simulink model "p3"  (R2020a)
settings: Solver=VariableStepAuto  StartTime=0.0  StopTime=10  RelTol=1e-3
model workspace (MAT data in the model file):
  A = Simulink.Parameter
  A.Value = 0.5792
  A.DataType = 'auto'
  A.Dimensions = [1 1]
  B = Simulink.Parameter
  B.Value = -1
  B.DataType = 'auto'
  B.Dimensions = [1 1]
  C = Simulink.Parameter
  C.Value = 1
  C.DataType = 'auto'
  C.Dimensions = [1 1]
  D = Simulink.Parameter
  D.Value = 0.1584
  D.DataType = 'auto'
  D.Dimensions = [1 1]
settings Model: Creator=007  LastModifiedBy=007

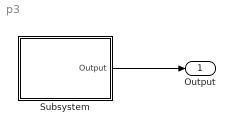
== system p3 ==
  Subsystem : Subsystem
  Output : Outport
  wires:
  Subsystem/1(Output) -> Output/1

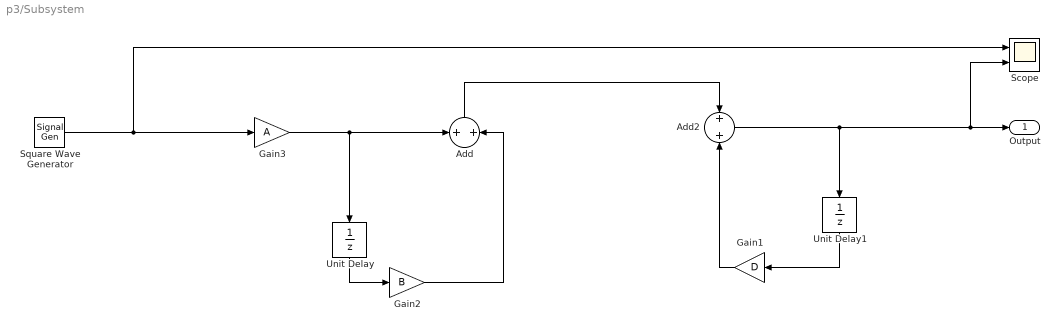
== system p3/Subsystem ==
  Add : Sum
  Add2 : Sum
  Gain1 : Gain  Gain=D
  Gain2 : Gain  Gain=B
  Gain3 : Gain  Gain=A
  Scope : Scope  NumInputPorts=2
  Square Wave Generator : SignalGenerator  WaveForm=square  Frequency=10  Units=rad/sec
  Unit Delay : UnitDelay  SampleTime=-1  HasFrameUpgradeWarning=on
  Unit Delay1 : UnitDelay  SampleTime=-1  HasFrameUpgradeWarning=on
  Output : Outport
  wires:
  Unit Delay/1 -> Gain2/1
  Unit Delay1/1 -> Gain1/1
  Add/1 -> Add2/1
  Gain3/1 -> Unit Delay/1, Add/1
  Gain1/1 -> Add2/2
  Add2/1 -> Unit Delay1/1, Scope/2, Output/1
  Square Wave Generator/1 -> Scope/1, Gain3/1
  Gain2/1 -> Add/2
